simulink model "Pure_Pursuit"  (R2020b)
settings: Solver=FixedStepAuto  StartTime=0.0  StopTime=50  RelTol=1e-3
undefined symbols (not defined in the file or in its folder): L, sampleTime
libraries: mobileRoboticsLib x2, robotalgslib x1
settings Model: EnablePacing=on  Creator=Tomas  LastModifiedBy=Tomas

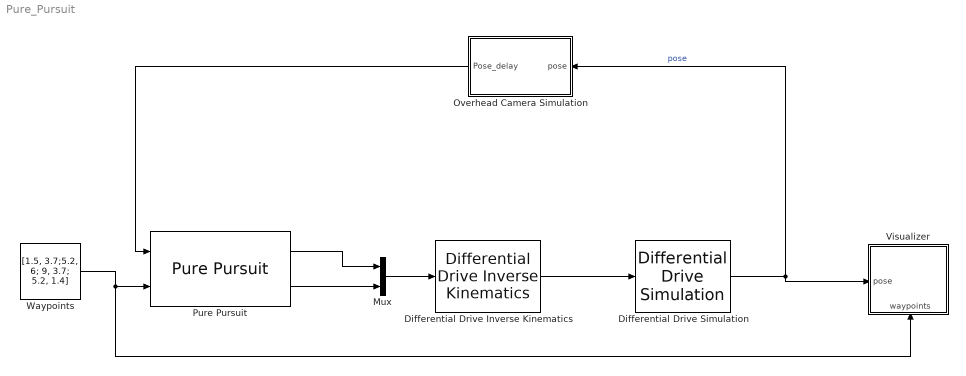
== system Pure_Pursuit ==
  Differential Drive Inverse Kinematics : mobileRoboticsLib/Kinematic Models/Differential Drive/Differential Drive Inverse Kinematics  wheelRadius=R  wheelBase=L
      settings: SourceProductName=Mobile Robotics Simulation Library
  Differential Drive Simulation : mobileRoboticsLib/Kinematic Models/Differential Drive/Differential Drive Simulation  wheelRadius=R  wheelBase=L  initX=1  initY=1  initAngle=0  Ts=sampleTime
      settings: SourceProductName=Mobile Robotics Simulation Library
  Mux : Mux  Inputs=2
  Overhead Camera Simulation : Subsystem
  Pure Pursuit : robotalgslib/Pure Pursuit  DesiredLinearVelocity=0.8  MaxAngularVelocity=1  LookaheadDistance=0.8  TargetDirPort=off  SimulateUsing=Code generation
  Visualizer : Subsystem
      settings: PortSchema="{\"entries\":[{\"content\":{\"sides\":[{\"content\":{\"connectorIds\":[\"In1\"]},\"type\":\"ConnectorPlacement.EquallySpacedRectSide\",\"uuid\":\"244d0762-dfc1-4b52-a6a1-a80beaccb9a2\"},{\"content\":{\"connectorIds\":[],\"side\":\"RIGHT\"},\"type\":\"ConnectorPlacement.EquallySpacedRectSide\",\"uuid\":\"1177407b-a167-4aa1-a3db-4054757a9ecb\"},{\"content\":{\"connectorIds\":[],\"side\":\"TOP\"},\"type\":\"ConnectorPlacement.EquallySpacedRectSide\",\"uuid\":\"a0f404aa-86c6-472b-9c46-22c4a2279521\"},{\"content\":{\"connectorIds\":[\"In2\"],\"side\":\"BOTTOM\"},\"type\":\"ConnectorPlacement.EquallySpacedRectSide\",\"uuid\":\"78b70b87-e4b1-4446-81a6-c2419c716c35\"},{\"content\":{\"connectorIds\":[],\"side\":\"HIDDEN\"},\"type\":\"ConnectorPlacement.EquallySpacedRectSide\",\"uuid\":\"2ba6edeb-1923-41ab-99af-1be794bc2de4\"}]},\"type\":\"ConnectorPlacement.EquallySpacedConnector\",\"uuid\":\"2f398c43-6025-4526-8334-cf398cbff666\"}],\"packageUris\":[\"http://schema.mathworks.com/mf0/Connector/R2020b\"],\"version\":\"1.0\"}"
  Waypoints : Constant  Value=[1.5, 3.7;5.2, 6; 9, 3.7; 5.2, 1.4]
  wires:
  Differential Drive Inverse Kinematics/1 -> Differential Drive Simulation/1
  Differential Drive Simulation/1 -> Overhead Camera Simulation/1(pose), Visualizer/1(pose)  "pose"
  Mux/1 -> Differential Drive Inverse Kinematics/1
  Pure Pursuit/1 -> Mux/1
  Pure Pursuit/2 -> Mux/2
  Waypoints/1 -> Visualizer/2(waypoints), Pure Pursuit/2
  Overhead Camera Simulation/1(Pose_delay) -> Pure Pursuit/1

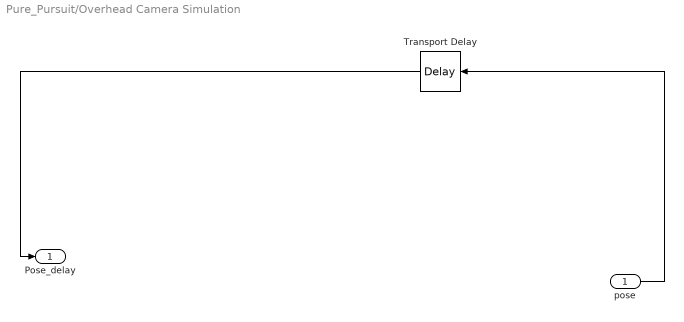
== system Pure_Pursuit/Overhead Camera Simulation ==
  pose : Inport
  Transport Delay : TransportDelay  DelayTime=0.1
  Pose_delay : Outport
  wires:
  pose/1 -> Transport Delay/1
  Transport Delay/1 -> Pose_delay/1

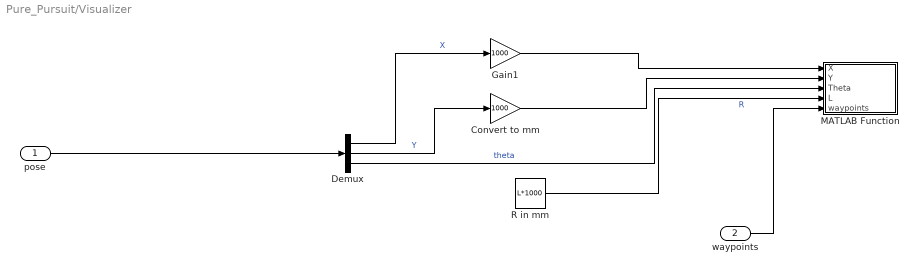
== system Pure_Pursuit/Visualizer ==
  pose : Inport
  waypoints : Inport  Port=2
  Convert to mm : Gain  Gain=1000
  Demux : Demux  Outputs=3
  Gain1 : Gain  Gain=1000
  MATLAB Function : MATLAB Function  TreatAsAtomicUnit=on
  R in mm : Constant  Value=L*1000
  wires:
  R in mm/1 -> MATLAB Function/4(L)  "R"
  Demux/2 -> Convert to mm/1  "Y"
  Convert to mm/1 -> MATLAB Function/2(Y)
  Demux/3 -> MATLAB Function/3(Theta)  "theta"
  Demux/1 -> Gain1/1  "X"
  Gain1/1 -> MATLAB Function/1(X)
  pose/1 -> Demux/1
  waypoints/1 -> MATLAB Function/5(waypoints)

== matlab function Pure_Pursuit/Visualizer/MATLAB Function ==
  data: X input; Y input; Theta input; L input; waypoints input
function fcn(X,Y,Theta, L, waypoints)
%% Robot Construction
% th = 0:pi/50:2*pi;
% RobotR = 100;
% xunit = L * cos(th) + X;
% yunit = L * sin(th) + Y;
robotRadius = L/2;
[xunit, yunit] = circle(X,Y,robotRadius);
% Robot Direction
RobotVector = 200;
VectorX = linspace(X,RobotVector*cos(Theta) + X);
VectorY = linspace(Y,RobotVector*sin(Theta) + Y);

%% middle Circle
[xcircle, ycircle] = circle(5200,3700,500);
%% Edge Coordinates
OuterEdgeX =[linspace(0,0) linspace(0,10400) linspace(10400,10400) linspace(10400,0)];
OuterEdgeY =[linspace(0,7400) linspace(7400,7400) linspace(7400,0) linspace(0,0)];   
InnerEdgeX = [linspace(400,400) linspace(400,10000) linspace(10000,10000) linspace(10000,400)];
InnerEdgeY = [linspace(400,7000) linspace(7000,7000) linspace(7000,400) linspace(400,400)]; 
PlayEdgeX = [linspace(700,700) linspace(700,9700) linspace(9700,9700) linspace(9700,700)];               
PlayEdgeY = [linspace(700,6700) linspace(6700,6700) linspace(6700,700) linspace(700,700)];
%% Horizontal Line of playground
x1 = linspace(700,9700);
y1 = linspace(3700,3700);
%% Vertical Line of playground
y2 = linspace(700,6700);
x2 = linspace(5200,5200);
%% Defence Area edges
defx0 =linspace(700,1700); defx1 = linspace(1700,1700);  defx2= linspace(1700,700); % 
defx00 =linspace(8700,9700); defx11 = linspace(8700,8700);  defx22= linspace(8700,9700);
defy0 =linspace(2700,2700);defy1 = linspace(2700,4700);  defy2= linspace(4700,4700);
Defx =[ defx0 defx1 defx2]; Defy = [defy0 defy1 defy2];
Defxx = [defx00 defx11 defx22]; Defyy = Defy;
%% Goal
Goalx0 =linspace(700,500); Goalx1 = linspace(500,500);  Goalx2= linspace(500,700);
Goaly0 =linspace(3200,3200); Goaly1 = linspace(3200,4200);  Goaly2= linspace(4200,4200);
Goalx =[ Goalx0 Goalx1 Goalx2]; Goaly = [Goaly0 Goaly1 Goaly2];
Goalx00 =linspace(9700,9900); Goalx11 = linspace(9900,9900);  Goalx22= linspace(9900,9700);
Goalxx =[ Goalx00 Goalx11 Goalx22]; Goalyy = Goaly;
% Waypoints utilities
waypoints=waypoints.*1000;
waypointsX = waypoints(:,1);
waypointsY = waypoints(:,2);
%% Plot

plot(x1,y1,'g',x2,y2,'g',Defx,Defy,'g',Defxx,Defyy,'g',Goalx,Goaly,'r',Goalxx,Goalyy,'r',...
   OuterEdgeX,OuterEdgeY,'g',InnerEdgeX,InnerEdgeY,'g',PlayEdgeX,PlayEdgeY,'g',...
    xcircle,ycircle,'g',waypointsX,waypointsY,'k+', xunit,yunit,'r',VectorX,VectorY,'b');
% plot(waypoints, 'k+');
xlim([0 10400])
ylim([0 7400])
